simulink model "stm32f4_delay_us_demo"  (Simulink 7.3)
settings: Solver=FixedStepDiscrete  SolverMode=SingleTasking  StartTime=0.0  StopTime=10.0  RelTol=1e-3
PreLoadFcn:
  | waijung.modelPreload; % Required for working with Waijung Blockset. Do not remove.
undefined symbols (not defined in the file): HSEOSC, Link, LQFP176, ST, STM32F417IG
libraries: stm32f4_io_lib x2, simulink x1, stm32f4_tim_lib x1, stm32f4_device_config_lib x1
CloseFcn:
  | waijung.modelClose; % Required for working with Waijung Blockset. Do not remove.
settings Model: Creator=Krisada  LastModifiedBy=Krisada
settings OptimizationCC: OptimizeModelRefInitCode=on  LifeSpan=1
settings HardwareCC: ProdEndianess=LittleEndian  ProdHWDeviceType=ARM Compatible->Cortex - M4  TargetEndianess=LittleEndian  TargetHWDeviceType=ARM Compatible->Cortex - M4
settings RTWCC: SystemTargetFile=stm32f4.tlc  GenerateMakefile=off  TemplateMakefile=ert_default_tmf  Description=STM32F4 Target  ProcessScript=stm32f4_make_rtw_hook
settings CodeAppCC: IgnoreCustomStorageClasses=off
settings STFCustomTargetCC: ModelReferenceCompliant=off  CombineOutputUpdateFcns=on  ERTCustomFileBanners=on  SupportContinuousTime=off  SupportNonInlinedSFcns=off  SystemTargetFile=stm32f4.tlc
settings ERTTargetCC: MultiwordLength=2048  ModelReferenceCompliant=off  ParMdlRefBuildCompliant=off  CompOptLevelCompliant=off  ERTFirstTimeCompliant=off  ModelStepFunctionPrototypeControlCompliant=off  CPPClassGenCompliant=off  ExtModeMexFile=noextcomm  InlinedParameterPlacement=NonHierarchical  ERTSrcFileBannerTemplate=stm32f4_code_template.cgt  ERTHdrFileBannerTemplate=stm32f4_code_template.cgt  ERTDataSrcFileTemplate=stm32f4_code_template.cgt  ERTDataHdrFileTemplate=stm32f4_code_template.cgt  ERTCustomFileTemplate=stm32f4_file_process.tlc

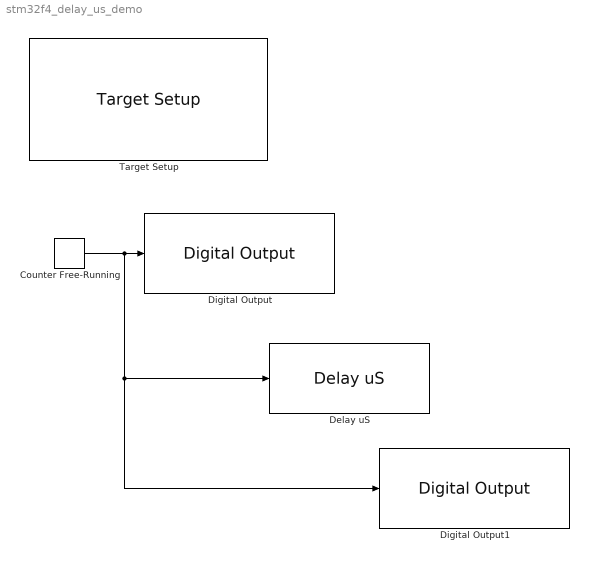
== system stm32f4_delay_us_demo ==
  Counter Free-Running : simulink/Sources/Counter Free-Running  SystemSampleTime=-1  NumBits=32  tsamp=2
  Delay uS : stm32f4_tim_lib/Delay uS  Priority=1  delaytime=1000000  enableinput=on  enableoutput=off  inputtypearray=[1 -1]  outputtypearray=[0]  sampletime=inf  sampletimestr=2  blockid=DelayuS
  Digital Output : stm32f4_io_lib/Digital Output  Priority=0  use_bitband=on  port=D  speed=100  porttype=Push Pull  porttypestr=PP  use_pin0=off  use_pin1=off  use_pin2=off  use_pin3=off  use_pin4=off  use_pin5=off  use_pin6=off  use_pin7=off  use_pin8=off  use_pin9=off  use_pin10=off  use_pin11=off  use_pin12=off  use_pin13=on  use_pin14=off  use_pin15=off  pinstr=GPIO_Pin_13  usedpinarray="[0  0  0  0  0  0  0  0  0  0  0  0  0  1  0  0]"  bitbandingstr="#define DigitalOutput_D13 Peripheral_BB(GPIOD->ODR, 13)  /* Output pin */"  sampletime=1  sampletimestr=1  blockid=DigitalOutput  enablecustomportlabel=off  globalinit=off  cinputportlabel=In1, In2  coutputportlabel=0
  Digital Output1 : stm32f4_io_lib/Digital Output  Priority=2  use_bitband=on  port=D  speed=100  porttype=Push Pull  porttypestr=PP  use_pin0=off  use_pin1=off  use_pin2=off  use_pin3=off  use_pin4=off  use_pin5=off  use_pin6=off  use_pin7=off  use_pin8=off  use_pin9=off  use_pin10=off  use_pin11=off  use_pin12=off  use_pin13=off  use_pin14=on  use_pin15=off  pinstr=GPIO_Pin_14  usedpinarray="[0  0  0  0  0  0  0  0  0  0  0  0  0  0  1  0]"  bitbandingstr="#define DigitalOutput1_D14 Peripheral_BB(GPIOD->ODR, 14)  /* Output pin */"  sampletime=1  sampletimestr=1  blockid=DigitalOutput1  enablecustomportlabel=off  globalinit=off  cinputportlabel=In1, In2  coutputportlabel=0
  Target Setup : stm32f4_device_config_lib/Target Setup  Priority=100  compiler=GNU ARM  previous_compiler=GNU ARM  mcu=STM32F417IG (LQFP176)  mcustr=STM32F417IG  clockconfig=HSEOSC-8MHz  system_stm32f4xx_c_path=F:\trunk\targets\stm32f4_target\stm32f4\utils\system_stm32f4xx_default\STM32F40_41xxx\hseosc8mhz  showmemoryconfiguration=off  stacksize=0x400  heapsize=0x200  enableautocompiledownload=on  fullchiperase=off  programmerinterface=ST-Link  editctrlstr=on  compilercontrolstr=$(patsubst %, -I%, .) -mcpu=cortex-m4 -mthumb -mthumb-interwork -mfloat-abi=hard -mfpu=fpv4-sp-d16 -ffast-math -Wall -Wextra -Ofast  assemblercontrolstr=$(patsubst %, -I%, .) -mcpu=cortex-m4 -mthumb -mthumb-interwork -mfloat-abi=hard -mfpu=fpv4-sp-d16 -ffast-math -Wall -Wextra -Ofast -Wa,-amhls=$(<:.s=.lst) -D__STACK_SIZE=$(STACK_SIZE) -D__HEAP_SIZE=$(HEAP_SIZE)  linkercontrolstr=-T$(LD_SCRIPT) -g -Wl,-Map=$(MAP),--cref,--no-warn-mismatch -mcpu=cortex-m4 -mthumb -mthumb-interwork -mfloat-abi=hard -mfpu=fpv4-sp-d16 -specs=nosys.specs  runafterdownload=on  execprofile=None  profileruart=1  profilerbaud=115200  profilertxpin=D8  profilerinitstr=0.01,168000000,1680000,115200,0  manualsetsampletime=off  sampletime=0.01  blockid=TargetSetup  systickreloadvalue=1680000  hseval=8000000  lastprofileruart=1  hclk=168000000  flashorigin=0x8000000  flashlength=1024k  ramorigin=0x20000000  ramlength=128k  useextram=off
  wires:
  Counter Free-Running/1 -> Digital Output/1, Digital Output1/1, Delay uS/1
